simulink model "Accelator_Padel_Sensor_Modeling"  (R2023a)
settings: Solver=FixedStepDiscrete  StartTime=0.0  StopTime=1  FixedStep=1e-3  RelTol=1e-3
libraries: simulink x3, pil_lib x1
settings Model: Creator=ItShop  LastModifiedBy=ItShop
settings OptimizationCC: DefaultParameterBehavior=Inlined  UseDivisionForNetSlopeComputation=on  GainParamInheritBuiltInType=on  UseFloatMulNetSlope=on  InlineInvariantSignals=on  PassReuseOutputArgsAs=Individual arguments  ZeroExternalMemoryAtStartup=off  ZeroInternalMemoryAtStartup=off  NoFixptDivByZeroProtection=on  EfficientFloat2IntCast=on  LifeSpan=1  OptimizeBlockOrder=speed  DifferentSizesBufferReuse=on  EfficientTunableParamExpr=on
settings DebuggingCC: ParameterTunabilityLossMsg=error
settings HardwareCC: ProdBitPerPointer=32  ProdBitPerSizeT=32  ProdBitPerPtrDiffT=32  ProdLargestAtomicInteger=Long  ProdLargestAtomicFloat=Double  ProdWordSize=32  ProdLongLongMode=on  ProdHWDeviceType=ARM Compatible->ARM Cortex-M
settings SFSimCC: MATLABDynamicMemAlloc=off
settings RTWCC: Description=Embedded Coder  SystemTargetFile=ert.tlc  TemplateMakefile=ert_default_tmf
settings CodeAppCC: ForceParamTrailComments=on  IgnoreCustomStorageClasses=off  OperatorAnnotations=on  SimulinkDataObjDesc=on  SFDataObjDesc=on  CustomSymbolStrGlobalVar=rt$N$M  CustomSymbolStrType=$N$M  CustomSymbolStrFcn=$N$M$F  CustomSymbolStrMacro=$N$M  InsertBlockDesc=on
settings ERTTargetCC: TargetLangStandard=C99 (ISO)  GenerateSampleERTMain=on  IncludeMdlTerminateFcn=off  CombineSignalStateStructs=on  SuppressErrorStatus=on  SupportAbsoluteTime=off  SupportComplex=off  InlinedParameterPlacement=NonHierarchical  ERTCustomFileTemplate=example_file_process.tlc  ERTFilePackagingFormat=CompactWithDataFile

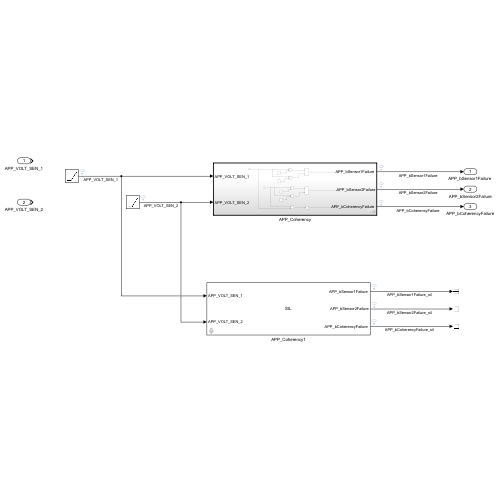
[thumbnail: Simulink's stored preview of the top-level diagram]
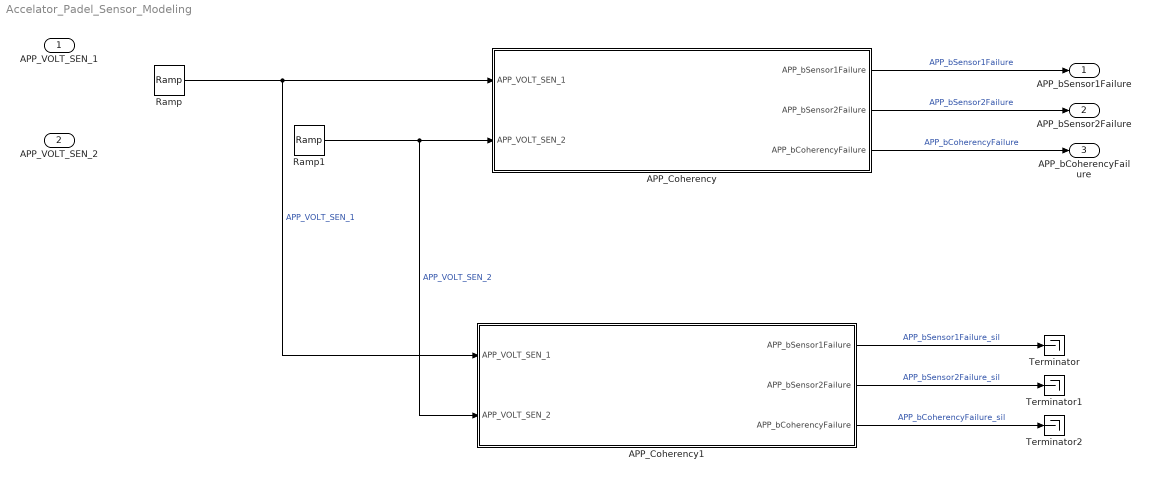
== system Accelator_Padel_Sensor_Modeling ==
  APP_VOLT_SEN_1 : Inport
  APP_VOLT_SEN_2 : Inport  Port=2
  APP_Coherency : Subsystem  TreatAsAtomicUnit=on
      settings: RTWSystemCode=Nonreusable function
  APP_Coherency1 : Subsystem  Tag=__SL_testing_harness_stub_  DialogController=pil_create_dialog  LoadFcn=|
      | try
      |    if ~strcmp(rtw.pil.getPILVersion, '9.14 (R2023a)_15')
      |       set_param(gcb, 'DialogController', '');
      |       set_param(gcb, 'DialogControllerArgs', '');
      |    end
      | catch e
      |       set_param(gcb, 'DialogController', '');
      |       set_param(gcb, 'DialogControllerArgs', '');
      | end
      mask help: PIL:pil:XILBlockMaskDesc
      mask Display: disp('SIL');
  Ramp : simulink/Sources/Ramp  slope=4  start=0  InitialOutput=.5
  Ramp1 : simulink/Sources/Ramp  slope=-4  start=0  InitialOutput=4.5
  Terminator : Terminator
  Terminator1 : Terminator
  Terminator2 : Terminator
  "APP_bSensor1Failure " : Outport
  APP_bSensor2Failure : Outport  Port=2
  " APP_bCoherencyFailure " : Outport  Port=3
  wires:
  APP_Coherency/1("APP_bSensor1Failure ") -> "APP_bSensor1Failure "/1  "APP_bSensor1Failure"
  APP_Coherency/2(APP_bSensor2Failure) -> APP_bSensor2Failure/1  "APP_bSensor2Failure"
  APP_Coherency/3(" APP_bCoherencyFailure ") -> " APP_bCoherencyFailure "/1  "APP_bCoherencyFailure"
  Ramp/1 -> APP_Coherency1/1(APP_VOLT_SEN_1), APP_Coherency/1(APP_VOLT_SEN_1)  "APP_VOLT_SEN_1"
  Ramp1/1 -> APP_Coherency1/2(APP_VOLT_SEN_2), APP_Coherency/2(APP_VOLT_SEN_2)  "APP_VOLT_SEN_2"
  APP_Coherency1/1("APP_bSensor1Failure ") -> Terminator/1  "APP_bSensor1Failure_sil"
  APP_Coherency1/2(APP_bSensor2Failure) -> Terminator1/1  "APP_bSensor2Failure_sil"
  APP_Coherency1/3(" APP_bCoherencyFailure ") -> Terminator2/1  "APP_bCoherencyFailure_sil"

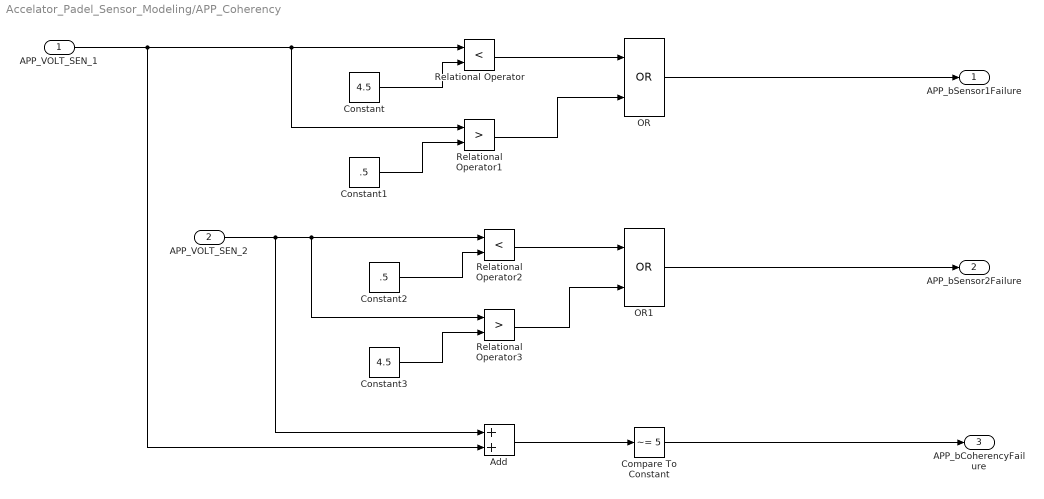
== system Accelator_Padel_Sensor_Modeling/APP_Coherency ==
  APP_VOLT_SEN_1 : Inport
  APP_VOLT_SEN_2 : Inport  Port=2
  Add : Sum
  Compare To Constant : simulink/Logic and Bit Operations/Compare To Constant  relop=~=  const=5  OutDataTypeStr=boolean
  Constant : Constant  Value=4.5
  Constant1 : Constant  Value=.5
  Constant2 : Constant  Value=.5
  Constant3 : Constant  Value=4.5
  OR : Logic  Operator=OR  AllPortsSameDT=off  OutDataTypeStr=boolean
  OR1 : Logic  Operator=OR  AllPortsSameDT=off  OutDataTypeStr=boolean
  Relational Operator : RelationalOperator  Operator=<  OutDataTypeStr=boolean  RndMeth=Simplest  InputSameDT=off
  Relational Operator1 : RelationalOperator  Operator=>  OutDataTypeStr=boolean  RndMeth=Simplest  InputSameDT=off
  Relational Operator2 : RelationalOperator  Operator=<  OutDataTypeStr=boolean  RndMeth=Simplest  InputSameDT=off
  Relational Operator3 : RelationalOperator  Operator=>  OutDataTypeStr=boolean  RndMeth=Simplest  InputSameDT=off
  "APP_bSensor1Failure " : Outport
  APP_bSensor2Failure : Outport  Port=2
  " APP_bCoherencyFailure " : Outport  Port=3
  wires:
  APP_VOLT_SEN_1/1 -> Add/2, Relational Operator1/1, Relational Operator/1
  Constant/1 -> Relational Operator/2
  Relational Operator/1 -> OR/1
  Constant1/1 -> Relational Operator1/2
  Relational Operator1/1 -> OR/2
  OR/1 -> "APP_bSensor1Failure "/1
  OR1/1 -> APP_bSensor2Failure/1
  Relational Operator3/1 -> OR1/2
  Constant3/1 -> Relational Operator3/2
  Relational Operator2/1 -> OR1/1
  Constant2/1 -> Relational Operator2/2
  APP_VOLT_SEN_2/1 -> Add/1, Relational Operator2/1, Relational Operator3/1
  Add/1 -> Compare To Constant/1
  Compare To Constant/1 -> " APP_bCoherencyFailure "/1

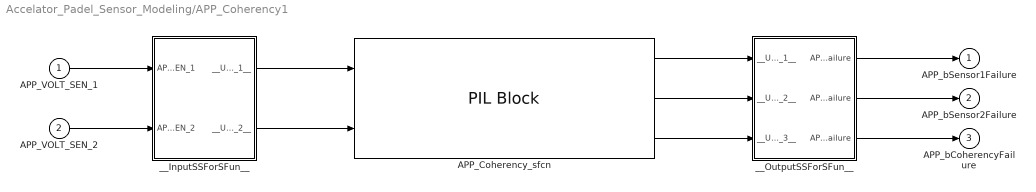
== system Accelator_Padel_Sensor_Modeling/APP_Coherency1 ==
  APP_VOLT_SEN_1 : Inport
  APP_VOLT_SEN_2 : Inport  Port=2
  APP_Coherency_sfcn : pil_lib/PIL Block  SimulationMode=SIL  IsTopModelPIL=off  CodeDir=APP_Coherency_ert_rtw  AnchorDir=E:\01_MBD Diploma\07_System Modeling Module\project  ConfigName=Software-in-the-Loop (SIL)  XrelIsTopModelCode=on  XrelIsReusable=off  XrelDWorkNames={}  XrelDWorkTypes={}  XrelModelArgVals={}  XrelOrderedParamNames={}
  __InputSSForSFun__ : Subsystem
  __OutputSSForSFun__ : Subsystem
  "APP_bSensor1Failure " : Outport
  APP_bSensor2Failure : Outport  Port=2
  " APP_bCoherencyFailure " : Outport  Port=3
  wires:
  __OutputSSForSFun__/3(" APP_bCoherencyFailure ") -> " APP_bCoherencyFailure "/1
  __OutputSSForSFun__/2(APP_bSensor2Failure) -> APP_bSensor2Failure/1
  __OutputSSForSFun__/1("APP_bSensor1Failure ") -> "APP_bSensor1Failure "/1
  APP_Coherency_sfcn/3 -> __OutputSSForSFun__/3(__UniqueInportName__3__)
  APP_Coherency_sfcn/2 -> __OutputSSForSFun__/2(__UniqueInportName__2__)
  APP_Coherency_sfcn/1 -> __OutputSSForSFun__/1(__UniqueInportName__1__)
  __InputSSForSFun__/2(__UniqueOutportName__2__) -> APP_Coherency_sfcn/2
  __InputSSForSFun__/1(__UniqueOutportName__1__) -> APP_Coherency_sfcn/1
  APP_VOLT_SEN_2/1 -> __InputSSForSFun__/2(APP_VOLT_SEN_2)
  APP_VOLT_SEN_1/1 -> __InputSSForSFun__/1(APP_VOLT_SEN_1)

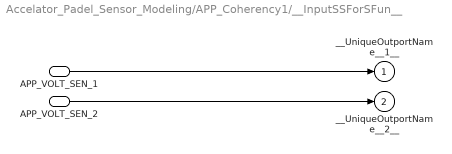
== system Accelator_Padel_Sensor_Modeling/APP_Coherency1/__InputSSForSFun__ ==
  APP_VOLT_SEN_1 : Inport
  APP_VOLT_SEN_2 : Inport  Port=2
  __UniqueOutportName__1__ : Outport
  __UniqueOutportName__2__ : Outport  Port=2
  wires:
  APP_VOLT_SEN_2/1 -> __UniqueOutportName__2__/1
  APP_VOLT_SEN_1/1 -> __UniqueOutportName__1__/1

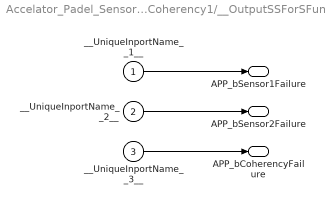
== system Accelator_Padel_Sensor_Modeling/APP_Coherency1/__OutputSSForSFun__ ==
  __UniqueInportName__1__ : Inport
  __UniqueInportName__2__ : Inport  Port=2
  __UniqueInportName__3__ : Inport  Port=3
  "APP_bSensor1Failure " : Outport
  APP_bSensor2Failure : Outport  Port=2
  " APP_bCoherencyFailure " : Outport  Port=3
  wires:
  __UniqueInportName__3__/1 -> " APP_bCoherencyFailure "/1
  __UniqueInportName__2__/1 -> APP_bSensor2Failure/1
  __UniqueInportName__1__/1 -> "APP_bSensor1Failure "/1
